simulink model "GS_model"  (R2018b)
settings: Solver=ode5  StartTime=0.0  StopTime=SimuStopTime  FixedStep=T_Simu  RelTol=1e-3
InitFcn:
  | Initial
undefined symbols (not defined in the file or in its folder): Aba10, Aba20, aeroCIP2006_S, aeroCIP2006_X, aeroCIP2006_Y, Agl0, Ass_kS, Ass_n1, Ass_n2, Ass_n3, Ass_n4, Ass_Noise, Ass_R, Ass_Resolution, Ass_TmOrder, AssA_Fix_Abs, AssB_Fix_Abs, AssC_Fix_Abs, AssD_Fix_Abs, AssE_Fix_Aps, AssF_Fix_Aps, C, c_max, c_min, Cd, CenterOfFigNX, CenterOfFigNY, CenterOfFigNZ, CenterOfFigP1, CenterOfFigP2, CenterOfFigPX, CenterOfFigPY, CenterOfFigPZ, Cmu, Crou, DEG2RAD, DiscIntNeverNeededParam, Eg_Dir, Eg_F, Eg_PrepareTime, Eg_r_L_L, Fw_Abf, Fw_Hmax, Fw_J, Fw_Spd0, Fw_Tmax, git_hash_BaseLine, git_hash_Project, Gnss_Noise_Pos, Gnss_Noise_Vel, Gnss_PropgationTime, GyroA_Fix_Abg, GyroA_Noise, GyroB_Fix_Abg, GyroB_Noise, GyroC_Fix_Abg, GyroC_Noise, GyroD_Fix_Abg, GyroD_Noise, h ... (+94)
libraries: simulink x308, sharedutil x46, aerolibutil x37, sharedtransform x31, vrlib x14, aerolibgravity2 x2
(part 14 of 20)

== system GS_model/Subsystem2/Subsystem/Actuator/Magnetorquer/Mt_MathModel/MtA3/Mag_CmdCal/>=<0 to 012 ==
  note: 1--正向
  note: 0
  note: 2--负向
  In1 : Inport
  Add1 : Sum  Inputs=+++
  Cast To Double : DataTypeConversion  OutDataTypeStr=double
  Cast To Double1 : DataTypeConversion  OutDataTypeStr=double
  Cast To Double2 : DataTypeConversion  OutDataTypeStr=double
  Compare To Zero : simulink/Logic and Bit Operations/Compare To Zero  relop=<  OutDataTypeStr=boolean
  Compare To Zero1 : simulink/Logic and Bit Operations/Compare To Zero  relop===  OutDataTypeStr=uint8
  Compare To Zero2 : simulink/Logic and Bit Operations/Compare To Zero  relop=>  OutDataTypeStr=boolean
  Constant1 : Constant
  Constant2 : Constant  Value=0
  Constant20 : Constant  Value=2
  Product1 : Product  SaturateOnIntegerOverflow=on  OutDataTypeStr=Inherit: Same as first input
  Product2 : Product  SaturateOnIntegerOverflow=on  OutDataTypeStr=Inherit: Same as first input
  Product6 : Product  SaturateOnIntegerOverflow=on  OutDataTypeStr=Inherit: Same as first input
  Out1 : Outport
  wires:
  Product1/1 -> Add1/2
  Product6/1 -> Add1/1
  Compare To Zero1/1 -> Cast To Double1/1
  Constant2/1 -> Product1/1
  In1/1 -> Compare To Zero2/1, Compare To Zero1/1, Compare To Zero/1
  Compare To Zero/1 -> Cast To Double/1
  Compare To Zero2/1 -> Cast To Double2/1
  Add1/1 -> Out1/1
  Cast To Double/1 -> Product6/2
  Cast To Double1/1 -> Product1/2
  Constant20/1 -> Product6/1
  Constant1/1 -> Product2/1
  Cast To Double2/1 -> Product2/2
  Product2/1 -> Add1/3

== system GS_model/Subsystem2/Subsystem/Actuator/Magnetorquer/Mt_MathModel/MtA4/Mag_CmdCal/55//AA to +//- ==
  note: 55H:正向
      | AAH:负向
  In1 : Inport
  Add1 : Sum  Inputs=|++
  Cast To Double : DataTypeConversion  OutDataTypeStr=double
  Cast To Double2 : DataTypeConversion  OutDataTypeStr=double
  Compare To Constant : simulink/Logic and Bit Operations/Compare To Constant  relop===  const=85  OutDataTypeStr=boolean
  Compare To Constant1 : simulink/Logic and Bit Operations/Compare To Constant  relop===  const=170  OutDataTypeStr=boolean
  Constant1 : Constant  Value=-1
  Constant20 : Constant
  Product2 : Product  SaturateOnIntegerOverflow=on  OutDataTypeStr=Inherit: Same as first input
  Product6 : Product  SaturateOnIntegerOverflow=on  OutDataTypeStr=Inherit: Same as first input
  Out1 : Outport
  wires:
  Constant1/1 -> Product2/2
  Cast To Double2/1 -> Product2/1
  Product2/1 -> Add1/2
  Constant20/1 -> Product6/1
  Cast To Double/1 -> Product6/2
  Add1/1 -> Out1/1
  Compare To Constant1/1 -> Cast To Double2/1
  Compare To Constant/1 -> Cast To Double/1
  In1/1 -> Compare To Constant1/1, Compare To Constant/1
  Product6/1 -> Add1/1

== system GS_model/Subsystem2/Subsystem/Actuator/Magnetorquer/Mt_MathModel/MtA4/Mag_CmdCal/>=<0 to 012 ==
  note: 2--负向
  note: 0
  note: 1--正向
  In1 : Inport
  Add1 : Sum  Inputs=+++
  Cast To Double : DataTypeConversion  OutDataTypeStr=double
  Cast To Double1 : DataTypeConversion  OutDataTypeStr=double
  Cast To Double2 : DataTypeConversion  OutDataTypeStr=double
  Compare To Zero : simulink/Logic and Bit Operations/Compare To Zero  relop=<  OutDataTypeStr=boolean
  Compare To Zero1 : simulink/Logic and Bit Operations/Compare To Zero  relop===  OutDataTypeStr=uint8
  Compare To Zero2 : simulink/Logic and Bit Operations/Compare To Zero  relop=>  OutDataTypeStr=boolean
  Constant1 : Constant
  Constant2 : Constant  Value=0
  Constant20 : Constant  Value=2
  Product1 : Product  SaturateOnIntegerOverflow=on  OutDataTypeStr=Inherit: Same as first input
  Product2 : Product  SaturateOnIntegerOverflow=on  OutDataTypeStr=Inherit: Same as first input
  Product6 : Product  SaturateOnIntegerOverflow=on  OutDataTypeStr=Inherit: Same as first input
  Out1 : Outport
  wires:
  Product2/1 -> Add1/3
  Cast To Double2/1 -> Product2/2
  Constant1/1 -> Product2/1
  Constant20/1 -> Product6/1
  Cast To Double1/1 -> Product1/2
  Cast To Double/1 -> Product6/2
  Add1/1 -> Out1/1
  Compare To Zero2/1 -> Cast To Double2/1
  Compare To Zero/1 -> Cast To Double/1
  In1/1 -> Compare To Zero/1, Compare To Zero1/1, Compare To Zero2/1
  Constant2/1 -> Product1/1
  Compare To Zero1/1 -> Cast To Double1/1
  Product6/1 -> Add1/1
  Product1/1 -> Add1/2

== system GS_model/Subsystem2/Subsystem/Actuator/Magnetorquer/Mt_MathModel/MtA5/Mag_CmdCal/55//AA to +//- ==
  note: 55H:正向
      | AAH:负向
  In1 : Inport
  Add1 : Sum  Inputs=|++
  Cast To Double : DataTypeConversion  OutDataTypeStr=double
  Cast To Double2 : DataTypeConversion  OutDataTypeStr=double
  Compare To Constant : simulink/Logic and Bit Operations/Compare To Constant  relop===  const=85  OutDataTypeStr=boolean
  Compare To Constant1 : simulink/Logic and Bit Operations/Compare To Constant  relop===  const=170  OutDataTypeStr=boolean
  Constant1 : Constant  Value=-1
  Constant20 : Constant
  Product2 : Product  SaturateOnIntegerOverflow=on  OutDataTypeStr=Inherit: Same as first input
  Product6 : Product  SaturateOnIntegerOverflow=on  OutDataTypeStr=Inherit: Same as first input
  Out1 : Outport
  wires:
  Product6/1 -> Add1/1
  In1/1 -> Compare To Constant/1, Compare To Constant1/1
  Compare To Constant/1 -> Cast To Double/1
  Compare To Constant1/1 -> Cast To Double2/1
  Add1/1 -> Out1/1
  Cast To Double/1 -> Product6/2
  Constant20/1 -> Product6/1
  Product2/1 -> Add1/2
  Cast To Double2/1 -> Product2/1
  Constant1/1 -> Product2/2

== system GS_model/Subsystem2/Subsystem/Actuator/Magnetorquer/Mt_MathModel/MtA5/Mag_CmdCal/>=<0 to 012 ==
  note: 1--正向
  note: 0
  note: 2--负向
  In1 : Inport
  Add1 : Sum  Inputs=+++
  Cast To Double : DataTypeConversion  OutDataTypeStr=double
  Cast To Double1 : DataTypeConversion  OutDataTypeStr=double
  Cast To Double2 : DataTypeConversion  OutDataTypeStr=double
  Compare To Zero : simulink/Logic and Bit Operations/Compare To Zero  relop=<  OutDataTypeStr=boolean
  Compare To Zero1 : simulink/Logic and Bit Operations/Compare To Zero  relop===  OutDataTypeStr=uint8
  Compare To Zero2 : simulink/Logic and Bit Operations/Compare To Zero  relop=>  OutDataTypeStr=boolean
  Constant1 : Constant
  Constant2 : Constant  Value=0
  Constant20 : Constant  Value=2
  Product1 : Product  SaturateOnIntegerOverflow=on  OutDataTypeStr=Inherit: Same as first input
  Product2 : Product  SaturateOnIntegerOverflow=on  OutDataTypeStr=Inherit: Same as first input
  Product6 : Product  SaturateOnIntegerOverflow=on  OutDataTypeStr=Inherit: Same as first input
  Out1 : Outport
  wires:
  Product1/1 -> Add1/2
  Product6/1 -> Add1/1
  Compare To Zero1/1 -> Cast To Double1/1
  Constant2/1 -> Product1/1
  In1/1 -> Compare To Zero2/1, Compare To Zero1/1, Compare To Zero/1
  Compare To Zero/1 -> Cast To Double/1
  Compare To Zero2/1 -> Cast To Double2/1
  Add1/1 -> Out1/1
  Cast To Double/1 -> Product6/2
  Cast To Double1/1 -> Product1/2
  Constant20/1 -> Product6/1
  Constant1/1 -> Product2/1
  Cast To Double2/1 -> Product2/2
  Product2/1 -> Add1/3

== system GS_model/Subsystem2/Subsystem/Actuator/Magnetorquer/Mt_MathModel/MtA6/Mag_CmdCal/55//AA to +//- ==
  note: 55H:正向
      | AAH:负向
  In1 : Inport
  Add1 : Sum  Inputs=|++
  Cast To Double : DataTypeConversion  OutDataTypeStr=double
  Cast To Double2 : DataTypeConversion  OutDataTypeStr=double
  Compare To Constant : simulink/Logic and Bit Operations/Compare To Constant  relop===  const=85  OutDataTypeStr=boolean
  Compare To Constant1 : simulink/Logic and Bit Operations/Compare To Constant  relop===  const=170  OutDataTypeStr=boolean
  Constant1 : Constant  Value=-1
  Constant20 : Constant
  Product2 : Product  SaturateOnIntegerOverflow=on  OutDataTypeStr=Inherit: Same as first input
  Product6 : Product  SaturateOnIntegerOverflow=on  OutDataTypeStr=Inherit: Same as first input
  Out1 : Outport
  wires:
  Constant1/1 -> Product2/2
  Cast To Double2/1 -> Product2/1
  Product2/1 -> Add1/2
  Constant20/1 -> Product6/1
  Cast To Double/1 -> Product6/2
  Add1/1 -> Out1/1
  Compare To Constant1/1 -> Cast To Double2/1
  Compare To Constant/1 -> Cast To Double/1
  In1/1 -> Compare To Constant1/1, Compare To Constant/1
  Product6/1 -> Add1/1

== system GS_model/Subsystem2/Subsystem/Actuator/Magnetorquer/Mt_MathModel/MtA6/Mag_CmdCal/>=<0 to 012 ==
  note: 2--负向
  note: 0
  note: 1--正向
  In1 : Inport
  Add1 : Sum  Inputs=+++
  Cast To Double : DataTypeConversion  OutDataTypeStr=double
  Cast To Double1 : DataTypeConversion  OutDataTypeStr=double
  Cast To Double2 : DataTypeConversion  OutDataTypeStr=double
  Compare To Zero : simulink/Logic and Bit Operations/Compare To Zero  relop=<  OutDataTypeStr=boolean
  Compare To Zero1 : simulink/Logic and Bit Operations/Compare To Zero  relop===  OutDataTypeStr=uint8
  Compare To Zero2 : simulink/Logic and Bit Operations/Compare To Zero  relop=>  OutDataTypeStr=boolean
  Constant1 : Constant
  Constant2 : Constant  Value=0
  Constant20 : Constant  Value=2
  Product1 : Product  SaturateOnIntegerOverflow=on  OutDataTypeStr=Inherit: Same as first input
  Product2 : Product  SaturateOnIntegerOverflow=on  OutDataTypeStr=Inherit: Same as first input
  Product6 : Product  SaturateOnIntegerOverflow=on  OutDataTypeStr=Inherit: Same as first input
  Out1 : Outport
  wires:
  Product2/1 -> Add1/3
  Cast To Double2/1 -> Product2/2
  Constant1/1 -> Product2/1
  Constant20/1 -> Product6/1
  Cast To Double1/1 -> Product1/2
  Cast To Double/1 -> Product6/2
  Add1/1 -> Out1/1
  Compare To Zero2/1 -> Cast To Double2/1
  Compare To Zero/1 -> Cast To Double/1
  In1/1 -> Compare To Zero/1, Compare To Zero1/1, Compare To Zero2/1
  Constant2/1 -> Product1/1
  Compare To Zero1/1 -> Cast To Double1/1
  Product6/1 -> Add1/1
  Product1/1 -> Add1/2

== system GS_model/Subsystem2/Subsystem/PhysicsModel/Environment/Air Torque Subsystem/satalite board/+Y SolarPanel/Compute press of sun radiation1 ==
  note: n
  "Abp " : Inport
  vs(b) : Inport  Port=2
  Fa' : Inport  Port=3
  Abs : Abs
  Dot Product : DotProduct  InputSameDT=on  OutDataTypeStr=Inherit: Inherit via internal rule
  Gain1 : Gain  Gain=S_P1  SaturateOnIntegerOverflow=on  OutDataTypeStr=Inherit: Same as input  ParamDataTypeStr=Inherit: Same as input
  Product1 : Product  Multiplication=Matrix(*)  SaturateOnIntegerOverflow=on  InputSameDT=on  OutDataTypeStr=Inherit: Same as first input
  Product3 : Product  SaturateOnIntegerOverflow=on  OutDataTypeStr=Inherit: Same as first input
  cons : Constant  Value=n_P1P
  "F_panel " : Outport
  wires:
  cons/1 -> Product1/2
  Abs/1 -> Gain1/1
  "Abp "/1 -> Product1/1
  Product1/1 -> Dot Product/2
  Dot Product/1 -> Abs/1
  Gain1/1 -> Product3/1
  Product3/1 -> "F_panel "/1
  Fa'/1 -> Product3/2
  vs(b)/1 -> Dot Product/1

== system GS_model/Subsystem2/Subsystem/PhysicsModel/Environment/Air Torque Subsystem/satalite board/+Y SolarPanel/compute centroi 1 ==
  Cent : Inport
  Abp_PY : Inport  Port=2
  Aba1 : Constant  Value=Aba10  VectorParams1D=off
  Product1 : Product  Multiplication=Matrix(*)  SaturateOnIntegerOverflow=on  InputSameDT=on  OutDataTypeStr=Inherit: Same as first input
  Product12 : Product  Multiplication=Matrix(*)  SaturateOnIntegerOverflow=on  InputSameDT=on  OutDataTypeStr=Inherit: Same as first input
  Sum2 : Sum  Inputs=|+-
  Sum3 : Sum  Inputs=+++  SaturateOnIntegerOverflow=on  InputSameDT=on  OutDataTypeStr=Inherit: Same as first input
  y3 : Constant  Value=CenterOfFigP1  VectorParams1D=off
  ·«°åa°²×°µãÎ»ÖÃ(L) : Constant  Value=r_L_a1_b  VectorParams1D=off
  ·«°åp°²×°µãÎ»ÖÃ(a0) : Constant  Value=r_a1_p1_a1  VectorParams1D=off
  r : Outport
  wires:
  Product12/1 -> Sum3/1
  Aba1/1 -> Product1/1
  ·«°åp°²×°µãÎ»ÖÃ(a0)/1 -> Product1/2
  Product1/1 -> Sum3/2
  y3/1 -> Product12/2
  ·«°åa°²×°µãÎ»ÖÃ(L)/1 -> Sum3/3
  Sum3/1 -> Sum2/1
  Abp_PY/1 -> Product12/1
  Cent/1 -> Sum2/2
  Sum2/1 -> r/1

== system GS_model/Subsystem2/Subsystem/PhysicsModel/Environment/Air Torque Subsystem/satalite board/-Y SolarPanel/Compute press of sun radiation ==
  note: n
  "Abp " : Inport
  vs(b) : Inport  Port=2
  Fa' : Inport  Port=3
  Abs : Abs
  Dot Product : DotProduct  InputSameDT=on  OutDataTypeStr=Inherit: Inherit via internal rule
  Gain1 : Gain  Gain=S_P2  SaturateOnIntegerOverflow=on  OutDataTypeStr=Inherit: Same as input  ParamDataTypeStr=Inherit: Same as input
  Product1 : Product  Multiplication=Matrix(*)  SaturateOnIntegerOverflow=on  InputSameDT=on  OutDataTypeStr=Inherit: Same as first input
  Product3 : Product  SaturateOnIntegerOverflow=on  OutDataTypeStr=Inherit: Same as first input
  cons : Constant  Value=n_P2P
  "F_panel " : Outport
  wires:
  cons/1 -> Product1/2
  Abs/1 -> Gain1/1
  "Abp "/1 -> Product1/1
  Product1/1 -> Dot Product/2
  Dot Product/1 -> Abs/1
  Gain1/1 -> Product3/1
  Product3/1 -> "F_panel "/1
  Fa'/1 -> Product3/2
  vs(b)/1 -> Dot Product/1

== system GS_model/Subsystem2/Subsystem/PhysicsModel/Environment/Air Torque Subsystem/satalite board/-Y SolarPanel/compute centroi 1 ==
  Cent : Inport
  Abp_NY : Inport  Port=2
  Aba1 : Constant  Value=Aba20  VectorParams1D=off
  Product1 : Product  Multiplication=Matrix(*)  SaturateOnIntegerOverflow=on  InputSameDT=on  OutDataTypeStr=Inherit: Same as first input
  Product12 : Product  Multiplication=Matrix(*)  SaturateOnIntegerOverflow=on  InputSameDT=on  OutDataTypeStr=Inherit: Same as first input
  Sum2 : Sum  Inputs=|+-
  Sum3 : Sum  Inputs=+++  SaturateOnIntegerOverflow=on  InputSameDT=on  OutDataTypeStr=Inherit: Same as first input
  y3 : Constant  Value=CenterOfFigP2  VectorParams1D=off
  ·«°åa°²×°µãÎ»ÖÃ(L) : Constant  Value=r_L_a2_b  VectorParams1D=off
  ·«°åp°²×°µãÎ»ÖÃ(a0) : Constant  Value=r_a2_p2_a2  VectorParams1D=off
  r : Outport
  wires:
  Sum2/1 -> r/1
  Cent/1 -> Sum2/2
  Abp_NY/1 -> Product12/1
  Sum3/1 -> Sum2/1
  ·«°åa°²×°µãÎ»ÖÃ(L)/1 -> Sum3/3
  y3/1 -> Product12/2
  Product1/1 -> Sum3/2
  ·«°åp°²×°µãÎ»ÖÃ(a0)/1 -> Product1/2
  Aba1/1 -> Product1/1
  Product12/1 -> Sum3/1

== system GS_model/Subsystem2/Subsystem/PhysicsModel/Environment/Air Torque Subsystem/satalite board/Torque from  board perpendicular to z axis /Compute press of sun radiation ==
  "[Vs]b_nor" : Inport
  Fa' : Inport  Port=2
  Board Orientation : Constant  Value=n_NZ  VectorParams1D=off
  Board Orientation1 : Constant  Value=n_PZ  VectorParams1D=off
  Board Orientation2 : Constant  Value=Szp_board  VectorParams1D=off
  Board Orientation3 : Constant  Value=Szn_board  VectorParams1D=off
  Dot Product : DotProduct  InputSameDT=on  OutDataTypeStr=Inherit: Inherit via internal rule
  Fcn : Fcn  Expr=u(3)
  Product3 : Product  Inputs=3  SaturateOnIntegerOverflow=on  OutDataTypeStr=Inherit: Same as first input
  Switch1 : Switch  SaturateOnIntegerOverflow=on  InputSameDT=on
  Switch2 : Switch  SaturateOnIntegerOverflow=on  InputSameDT=on
  Fz : Outport
  wires:
  Board Orientation1/1 -> Switch2/1
  Board Orientation/1 -> Switch2/3
  Fcn/1 -> Switch2/2
  "[Vs]b_nor"/1 -> Switch1/2, Fcn/1, Dot Product/1
  Switch2/1 -> Dot Product/2
  Product3/1 -> Fz/1
  Dot Product/1 -> Product3/2
  Fa'/1 -> Product3/3
  Board Orientation3/1 -> Switch1/3
  Board Orientation2/1 -> Switch1/1
  Switch1/1 -> Product3/1

== system GS_model/Subsystem2/Subsystem/PhysicsModel/Environment/Air Torque Subsystem/satalite board/Torque from  board perpendicular to z axis /compute centroi 1 ==
  Orientation : Inport
  Cent : Inport  Port=2
  Fcn : Fcn  Expr=u(3)
  Sum2 : Sum  Inputs=|+-
  Switch1 : Switch  SaturateOnIntegerOverflow=on  InputSameDT=on
  y2 : Constant  Value=CenterOfFigNZ  VectorParams1D=off
  y3 : Constant  Value=CenterOfFigPZ  VectorParams1D=off
  r_z : Outport
  wires:
  Sum2/1 -> r_z/1
  y3/1 -> Switch1/1
  y2/1 -> Switch1/3
  Fcn/1 -> Switch1/2
  Orientation/1 -> Fcn/1
  Cent/1 -> Sum2/2
  Switch1/1 -> Sum2/1

== system GS_model/Subsystem2/Subsystem/PhysicsModel/Environment/Air Torque Subsystem/satalite board/Torque from board perpendicular to x axis/Compute press of sun radiation ==
  note: S
  Vs(b) : Inport
  Fa' : Inport  Port=2
  Board Orientation : Constant  Value=n_NX  VectorParams1D=off
  Board Orientation1 : Constant  Value=n_PX  VectorParams1D=off
  Board Orientation2 : Constant  Value=Sx_board  VectorParams1D=off
  Dot Product : DotProduct  InputSameDT=on  OutDataTypeStr=Inherit: Inherit via internal rule
  Fcn : Fcn  Expr=u(1)
  Product3 : Product  Inputs=3  SaturateOnIntegerOverflow=on  OutDataTypeStr=Inherit: Same as first input
  Switch2 : Switch  SaturateOnIntegerOverflow=on  InputSameDT=on
  Fx : Outport
  wires:
  Board Orientation1/1 -> Switch2/1
  Board Orientation/1 -> Switch2/3
  Fcn/1 -> Switch2/2
  Switch2/1 -> Dot Product/2
  Vs(b)/1 -> Fcn/1, Dot Product/1
  Product3/1 -> Fx/1
  Dot Product/1 -> Product3/2
  Board Orientation2/1 -> Product3/1
  Fa'/1 -> Product3/3

== system GS_model/Subsystem2/Subsystem/PhysicsModel/Environment/Air Torque Subsystem/satalite board/Torque from board perpendicular to x axis/compute centroi 1 ==
  Orientation : Inport
  Cent : Inport  Port=2
  Fcn : Fcn  Expr=u(1)
  Sum2 : Sum  Inputs=|+-
  Switch1 : Switch  SaturateOnIntegerOverflow=on  InputSameDT=on
  y2 : Constant  Value=CenterOfFigNX  VectorParams1D=off
  y3 : Constant  Value=CenterOfFigPX  VectorParams1D=off
  r_x : Outport
  wires:
  Sum2/1 -> r_x/1
  y3/1 -> Switch1/1
  y2/1 -> Switch1/3
  Fcn/1 -> Switch1/2
  Orientation/1 -> Fcn/1
  Cent/1 -> Sum2/2
  Switch1/1 -> Sum2/1

== system GS_model/Subsystem2/Subsystem/PhysicsModel/Environment/Air Torque Subsystem/satalite board/Torque from board perpendicular to y axis/Compute press of sun radiation ==
  note: S
  vs(b) : Inport
  Fa' : Inport  Port=2
  Dot Product : DotProduct  InputSameDT=on  OutDataTypeStr=Inherit: Inherit via internal rule
  Fcn : Fcn  Expr=u(2)
  Product1 : Product  Inputs=3  SaturateOnIntegerOverflow=on  OutDataTypeStr=Inherit: Same as first input
  Switch2 : Switch  SaturateOnIntegerOverflow=on  InputSameDT=on
  x1 : Constant  Value=Sy_board  VectorParams1D=off
  x2 : Constant  Value=n_PY  VectorParams1D=off
  x3 : Constant  Value=n_NY  VectorParams1D=off
  Fy : Outport
  wires:
  x2/1 -> Switch2/1
  Fcn/1 -> Switch2/2
  vs(b)/1 -> Fcn/1, Dot Product/1
  Switch2/1 -> Dot Product/2
  Product1/1 -> Fy/1
  Dot Product/1 -> Product1/2
  x1/1 -> Product1/1
  Fa'/1 -> Product1/3
  x3/1 -> Switch2/3

== system GS_model/Subsystem2/Subsystem/PhysicsModel/Environment/Air Torque Subsystem/satalite board/Torque from board perpendicular to y axis/compute centroi 1 ==
  Orientation : Inport
  Cent : Inport  Port=2
  Fcn : Fcn  Expr=u(2)
  Sum2 : Sum  Inputs=|+-
  Switch1 : Switch  SaturateOnIntegerOverflow=on  InputSameDT=on
  y2 : Constant  Value=CenterOfFigNY  VectorParams1D=off
  y3 : Constant  Value=CenterOfFigPY  VectorParams1D=off
  r_y : Outport
  wires:
  Sum2/1 -> r_y/1
  y3/1 -> Switch1/1
  y2/1 -> Switch1/3
  Fcn/1 -> Switch1/2
  Orientation/1 -> Fcn/1
  Cent/1 -> Sum2/2
  Switch1/1 -> Sum2/1

== system GS_model/Subsystem2/Subsystem/PhysicsModel/Environment/Sun  press torque/Sun  press torque2/Sun  press torque/+Y SunPanel ==
  Sun(b) : Inport
  Cent : Inport  Port=2
  Abp : Inport  Port=3
  TC_SunPressCoeff : Inport  Port=4
  3x3 Cross Product : sharedutil/3x3 Cross Product  aMode=aMode
      settings: SourceProductBaseCode=AE,PW,MT,VE,VP
  Compute press of sun radiation : Subsystem  TreatAsAtomicUnit=on
  Product1 : Product  Multiplication=Matrix(*)  SaturateOnIntegerOverflow=on  InputSameDT=on  OutDataTypeStr=Inherit: Same as first input
  Product2 : Product  Multiplication=Matrix(*)  SaturateOnIntegerOverflow=on  InputSameDT=on  OutDataTypeStr=Inherit: Same as first input
  compute centroi 1 : Subsystem  TreatAsAtomicUnit=on
  transpose : Math  Operator=transpose  SaturateOnIntegerOverflow=on
  T : Outport
  F : Outport  Port=2
  wires:
  compute centroi 1/1(r) -> 3x3 Cross Product/1
  Product1/1 -> F/1, 3x3 Cross Product/2
  Compute press of sun radiation/1(F(p)) -> Product1/2
  Product2/1 -> Compute press of sun radiation/1(Sun(p))
  Abp/1 -> compute centroi 1/2(Abp_PY), transpose/1, Product1/1
  Sun(b)/1 -> Product2/2
  transpose/1 -> Product2/1
  Cent/1 -> compute centroi 1/1(Cent)
  3x3 Cross Product/1 -> T/1
  TC_SunPressCoeff/1 -> Compute press of sun radiation/2(TC_SunPressCoeff)

== system GS_model/Subsystem2/Subsystem/PhysicsModel/Environment/Sun  press torque/Sun  press torque2/Sun  press torque/-Y SunPanel ==
  Sun(b) : Inport
  Cent : Inport  Port=2
  Abp : Inport  Port=3
  TC_SunPressCoeff : Inport  Port=4
  3x3 Cross Product : sharedutil/3x3 Cross Product  aMode=aMode
      settings: SourceProductBaseCode=AE,PW,MT,VE,VP
  Compute press of sun radiation : Subsystem  TreatAsAtomicUnit=on
  Product1 : Product  Multiplication=Matrix(*)  SaturateOnIntegerOverflow=on  InputSameDT=on  OutDataTypeStr=Inherit: Same as first input
  Product2 : Product  Multiplication=Matrix(*)  SaturateOnIntegerOverflow=on  InputSameDT=on  OutDataTypeStr=Inherit: Same as first input
  compute centroi 1 : Subsystem  TreatAsAtomicUnit=on
  transpose : Math  Operator=transpose  SaturateOnIntegerOverflow=on
  T : Outport
  F : Outport  Port=2
  wires:
  3x3 Cross Product/1 -> T/1
  Cent/1 -> compute centroi 1/1(Cent)
  transpose/1 -> Product2/1
  Sun(b)/1 -> Product2/2
  Abp/1 -> Product1/1, transpose/1, compute centroi 1/2(Abp_NY)
  Product2/1 -> Compute press of sun radiation/1(Sun(p))
  Compute press of sun radiation/1(F(p)) -> Product1/2
  Product1/1 -> 3x3 Cross Product/2, F/1
  compute centroi 1/1(r) -> 3x3 Cross Product/1
  TC_SunPressCoeff/1 -> Compute press of sun radiation/2(TC_SunPressCoeff)

== system GS_model/Subsystem2/Subsystem/PhysicsModel/Environment/Sun  press torque/Sun  press torque2/Sun  press torque/Torque from   satalite board ==
  SunOrientation : Inport
  Cent : Inport  Port=2
  TC_SunPressCoeff : Inport  Port=3
  Sum : Sum  Inputs=+++
  Sum1 : Sum  Inputs=+++
  "Torque from  board perpendicular to z axis " : Subsystem  TreatAsAtomicUnit=on
  Torque from board perpendicular to x axis : Subsystem  TreatAsAtomicUnit=on
  Torque from board perpendicular to y axis : Subsystem  TreatAsAtomicUnit=on
  T_board : Outport
  F_board : Outport  Port=2
  wires:
  Sum1/1 -> F_board/1
  Sum/1 -> T_board/1
  Torque from board perpendicular to x axis/2(Fx) -> Sum1/1
  Torque from board perpendicular to y axis/2(Fy) -> Sum1/2
  "Torque from  board perpendicular to z axis "/2(Fz) -> Sum1/3
  "Torque from  board perpendicular to z axis "/1(Tz) -> Sum/3
  Torque from board perpendicular to x axis/1(Tx) -> Sum/1
  Torque from board perpendicular to y axis/1(Ty) -> Sum/2
  SunOrientation/1 -> "Torque from  board perpendicular to z axis "/1(Sun Orientation), Torque from board perpendicular to y axis/1(Sun Orientation), Torque from board perpendicular to x axis/1(Sun Orientation)
  Cent/1 -> "Torque from  board perpendicular to z axis "/2(Cent), Torque from board perpendicular to y axis/2(Cent), Torque from board perpendicular to x axis/2(Cent)
  TC_SunPressCoeff/1 -> "Torque from  board perpendicular to z axis "/3(TC_SunPressCoeff), Torque from board perpendicular to y axis/3(TC_SunPressCoeff), Torque from board perpendicular to x axis/3(TC_SunPressCoeff)

== system GS_model/Subsystem2/Subsystem/Sensor/Ass/BodyAss(A&B&C&D)Model/Subsystem/AssErrModel/AssErrSet ==
  note: Switch
  note: Period
  note: AmpCoff
  note: Switch
  note: AmpCoff
  AssCur : Inport
  TC_AssErr_Constant : Inport  Port=2
  TC_AssErr_WildValue : Inport  Port=3
  TC_AssErr_Jump : Inport  Port=4
  TC_StErr_Wave : Inport  Port=5
  AssErrSet_Constant : Subsystem
  AssErrSet_Jump : Subsystem
  AssErrSet_Wave : Subsystem
  AssErrSet_WildValue : Subsystem
  Demux : Demux  Outputs=2
  Demux1 : Demux  Outputs=3
  JumpSet : Constant  Value=0.04
  Terminator : Terminator
  WaveSet : SignalGenerator  WaveForm=square
  WildValueSet : Constant  Value=0.09
  TM_Ass_Cur : Outport
  wires:
  TC_StErr_Wave/1 -> Demux/1
  TC_AssErr_Jump/1 -> Demux1/1
  Demux1/2 -> Terminator/1
  WildValueSet/1 -> AssErrSet_WildValue/2(ErrValue)
  TC_AssErr_WildValue/1 -> AssErrSet_WildValue/3(ErrSwitch)
  TC_AssErr_Constant/1 -> AssErrSet_Constant/1(ErrSwitch)
  AssCur/1 -> AssErrSet_Constant/2(Ass_in)
  AssErrSet_Constant/1(Ass_out) -> AssErrSet_WildValue/1(Ass_in)
  AssErrSet_WildValue/1(Ass_out) -> AssErrSet_Jump/1(Ass_in)
  Demux1/1 -> AssErrSet_Jump/3(ErrSwitch)
  Demux1/3 -> AssErrSet_Jump/4(AssJumpErrAmpCoff)
  JumpSet/1 -> AssErrSet_Jump/2(ErrValue)
  AssErrSet_Jump/1(Ass_out) -> AssErrSet_Wave/1(Ass_in)
  AssErrSet_Wave/1(Ass_out) -> TM_Ass_Cur/1
  WaveSet/1 -> AssErrSet_Wave/2(ErrValue)
  Demux/1 -> AssErrSet_Wave/3(ErrSwitch)
  Demux/2 -> AssErrSet_Wave/4(AssWaveErrAmpCoff)

== system GS_model/Subsystem2/Subsystem/Sensor/Ass/BodyAss(A&B&C&D)Model/Subsystem/AssErrModel/If Action Subsystem ==
  In1 : Inport
  Action Port : ActionPort  ActionType=then
  Out1 : Outport
  wires:
  In1/1 -> Out1/1

== system GS_model/Subsystem2/Subsystem/Sensor/Ass/BodyAss(A&B&C&D)Model/Subsystem/AssErrModel/If Action Subsystem1 ==
  In1 : Inport
  Action Port : ActionPort  ActionType=else
  Out1 : Outport
  wires:
  In1/1 -> Out1/1

== system GS_model/Subsystem2/Subsystem/Sensor/Ass/BodyAss(A&B&C&D)Model/Subsystem/AssErrModel/Triggered Subsystem1 ==
  In1 : Inport
  Enable : EnablePort
  Out1 : Outport  InitialOutput=0
  wires:
  In1/1 -> Out1/1

== system GS_model/Subsystem2/Subsystem/Sensor/Ass/BodyAss(A&B&C&D)Model/Subsystem/AssErrModel/Triggered Subsystem2 ==
  In1 : Inport
  Enable : EnablePort
  Out1 : Outport  InitialOutput=0
  wires:
  In1/1 -> Out1/1

== system GS_model/Subsystem2/Subsystem/Sensor/Ass/BodyAss(A&B&C&D)Model/Subsystem/AssErrModel/Triggered Subsystem3 ==
  In1 : Inport
  Enable : EnablePort
  Out1 : Outport  InitialOutput=0
  wires:
  In1/1 -> Out1/1

== system GS_model/Subsystem2/Subsystem/Sensor/Ass/BodyAss(A&B&C&D)Model/Subsystem/AssErrModel/Triggered Subsystem4 ==
  In1 : Inport
  Enable : EnablePort
  Out1 : Outport  InitialOutput=0
  wires:
  In1/1 -> Out1/1

== system GS_model/Subsystem2/Subsystem/Sensor/Ass/BodyAss(A&B&C&D)Model/Subsystem/AssErrModel/Triggered Subsystem5 ==
  In1 : Inport
  Enable : EnablePort
  Out1 : Outport  InitialOutput=0
  wires:
  In1/1 -> Out1/1

== system GS_model/Subsystem2/Subsystem/Sensor/Ass/BodyAss(A&B&C&D)Model/Subsystem1/AssErrModel/AssErrSet ==
  note: AmpCoff
  note: Switch
  note: AmpCoff
  note: Period
  note: Switch
  AssCur : Inport
  TC_AssErr_Constant : Inport  Port=2
  TC_AssErr_WildValue : Inport  Port=3
  TC_AssErr_Jump : Inport  Port=4
  TC_StErr_Wave : Inport  Port=5
  AssErrSet_Constant : Subsystem
  AssErrSet_Jump : Subsystem
  AssErrSet_Wave : Subsystem
  AssErrSet_WildValue : Subsystem
  Demux : Demux  Outputs=2
  Demux1 : Demux  Outputs=3
  JumpSet : Constant  Value=0.04
  Terminator : Terminator
  WaveSet : SignalGenerator  WaveForm=square
  WildValueSet : Constant  Value=0.09
  TM_Ass_Cur : Outport
  wires:
  Demux/2 -> AssErrSet_Wave/4(AssWaveErrAmpCoff)
  Demux/1 -> AssErrSet_Wave/3(ErrSwitch)
  WaveSet/1 -> AssErrSet_Wave/2(ErrValue)
  AssErrSet_Wave/1(Ass_out) -> TM_Ass_Cur/1
  AssErrSet_Jump/1(Ass_out) -> AssErrSet_Wave/1(Ass_in)
  JumpSet/1 -> AssErrSet_Jump/2(ErrValue)
  Demux1/3 -> AssErrSet_Jump/4(AssJumpErrAmpCoff)
  Demux1/1 -> AssErrSet_Jump/3(ErrSwitch)
  AssErrSet_WildValue/1(Ass_out) -> AssErrSet_Jump/1(Ass_in)
  AssErrSet_Constant/1(Ass_out) -> AssErrSet_WildValue/1(Ass_in)
  AssCur/1 -> AssErrSet_Constant/2(Ass_in)
  TC_AssErr_Constant/1 -> AssErrSet_Constant/1(ErrSwitch)
  TC_AssErr_WildValue/1 -> AssErrSet_WildValue/3(ErrSwitch)
  WildValueSet/1 -> AssErrSet_WildValue/2(ErrValue)
  Demux1/2 -> Terminator/1
  TC_AssErr_Jump/1 -> Demux1/1
  TC_StErr_Wave/1 -> Demux/1

== system GS_model/Subsystem2/Subsystem/Sensor/Ass/BodyAss(A&B&C&D)Model/Subsystem1/AssErrModel/If Action Subsystem ==
  In1 : Inport
  Action Port : ActionPort  ActionType=then
  Out1 : Outport
  wires:
  In1/1 -> Out1/1

== system GS_model/Subsystem2/Subsystem/Sensor/Ass/BodyAss(A&B&C&D)Model/Subsystem1/AssErrModel/If Action Subsystem1 ==
  In1 : Inport
  Action Port : ActionPort  ActionType=else
  Out1 : Outport
  wires:
  In1/1 -> Out1/1

== system GS_model/Subsystem2/Subsystem/Sensor/Ass/BodyAss(A&B&C&D)Model/Subsystem1/AssErrModel/Triggered Subsystem1 ==
  In1 : Inport
  Enable : EnablePort
  Out1 : Outport  InitialOutput=0
  wires:
  In1/1 -> Out1/1

== system GS_model/Subsystem2/Subsystem/Sensor/Ass/BodyAss(A&B&C&D)Model/Subsystem1/AssErrModel/Triggered Subsystem2 ==
  In1 : Inport
  Enable : EnablePort
  Out1 : Outport  InitialOutput=0
  wires:
  In1/1 -> Out1/1

== system GS_model/Subsystem2/Subsystem/Sensor/Ass/BodyAss(A&B&C&D)Model/Subsystem1/AssErrModel/Triggered Subsystem3 ==
  In1 : Inport
  Enable : EnablePort
  Out1 : Outport  InitialOutput=0
  wires:
  In1/1 -> Out1/1

== system GS_model/Subsystem2/Subsystem/Sensor/Ass/BodyAss(A&B&C&D)Model/Subsystem1/AssErrModel/Triggered Subsystem4 ==
  In1 : Inport
  Enable : EnablePort
  Out1 : Outport  InitialOutput=0
  wires:
  In1/1 -> Out1/1

== system GS_model/Subsystem2/Subsystem/Sensor/Ass/BodyAss(A&B&C&D)Model/Subsystem1/AssErrModel/Triggered Subsystem5 ==
  In1 : Inport
  Enable : EnablePort
  Out1 : Outport  InitialOutput=0
  wires:
  In1/1 -> Out1/1

== system GS_model/Subsystem2/Subsystem/Sensor/Ass/BodyAss(A&B&C&D)Model/Subsystem2/AssErrModel/AssErrSet ==
  note: Switch
  note: Period
  note: AmpCoff
  note: Switch
  note: AmpCoff
  AssCur : Inport
  TC_AssErr_Constant : Inport  Port=2
  TC_AssErr_WildValue : Inport  Port=3
  TC_AssErr_Jump : Inport  Port=4
  TC_StErr_Wave : Inport  Port=5
  AssErrSet_Constant : Subsystem
  AssErrSet_Jump : Subsystem
  AssErrSet_Wave : Subsystem
  AssErrSet_WildValue : Subsystem
  Demux : Demux  Outputs=2
  Demux1 : Demux  Outputs=3
  JumpSet : Constant  Value=0.04
  Terminator : Terminator
  WaveSet : SignalGenerator  WaveForm=square
  WildValueSet : Constant  Value=0.09
  TM_Ass_Cur : Outport
  wires:
  TC_StErr_Wave/1 -> Demux/1
  TC_AssErr_Jump/1 -> Demux1/1
  Demux1/2 -> Terminator/1
  WildValueSet/1 -> AssErrSet_WildValue/2(ErrValue)
  TC_AssErr_WildValue/1 -> AssErrSet_WildValue/3(ErrSwitch)
  TC_AssErr_Constant/1 -> AssErrSet_Constant/1(ErrSwitch)
  AssCur/1 -> AssErrSet_Constant/2(Ass_in)
  AssErrSet_Constant/1(Ass_out) -> AssErrSet_WildValue/1(Ass_in)
  AssErrSet_WildValue/1(Ass_out) -> AssErrSet_Jump/1(Ass_in)
  Demux1/1 -> AssErrSet_Jump/3(ErrSwitch)
  Demux1/3 -> AssErrSet_Jump/4(AssJumpErrAmpCoff)
  JumpSet/1 -> AssErrSet_Jump/2(ErrValue)
  AssErrSet_Jump/1(Ass_out) -> AssErrSet_Wave/1(Ass_in)
  AssErrSet_Wave/1(Ass_out) -> TM_Ass_Cur/1
  WaveSet/1 -> AssErrSet_Wave/2(ErrValue)
  Demux/1 -> AssErrSet_Wave/3(ErrSwitch)
  Demux/2 -> AssErrSet_Wave/4(AssWaveErrAmpCoff)

== system GS_model/Subsystem2/Subsystem/Sensor/Ass/BodyAss(A&B&C&D)Model/Subsystem2/AssErrModel/If Action Subsystem ==
  In1 : Inport
  Action Port : ActionPort  ActionType=then
  Out1 : Outport
  wires:
  In1/1 -> Out1/1

== system GS_model/Subsystem2/Subsystem/Sensor/Ass/BodyAss(A&B&C&D)Model/Subsystem2/AssErrModel/If Action Subsystem1 ==
  In1 : Inport
  Action Port : ActionPort  ActionType=else
  Out1 : Outport
  wires:
  In1/1 -> Out1/1

== system GS_model/Subsystem2/Subsystem/Sensor/Ass/BodyAss(A&B&C&D)Model/Subsystem2/AssErrModel/Triggered Subsystem1 ==
  In1 : Inport
  Enable : EnablePort
  Out1 : Outport  InitialOutput=0
  wires:
  In1/1 -> Out1/1

== system GS_model/Subsystem2/Subsystem/Sensor/Ass/BodyAss(A&B&C&D)Model/Subsystem2/AssErrModel/Triggered Subsystem2 ==
  In1 : Inport
  Enable : EnablePort
  Out1 : Outport  InitialOutput=0
  wires:
  In1/1 -> Out1/1

== system GS_model/Subsystem2/Subsystem/Sensor/Ass/BodyAss(A&B&C&D)Model/Subsystem2/AssErrModel/Triggered Subsystem3 ==
  In1 : Inport
  Enable : EnablePort
  Out1 : Outport  InitialOutput=0
  wires:
  In1/1 -> Out1/1

== system GS_model/Subsystem2/Subsystem/Sensor/Ass/BodyAss(A&B&C&D)Model/Subsystem2/AssErrModel/Triggered Subsystem4 ==
  In1 : Inport
  Enable : EnablePort
  Out1 : Outport  InitialOutput=0
  wires:
  In1/1 -> Out1/1

== system GS_model/Subsystem2/Subsystem/Sensor/Ass/BodyAss(A&B&C&D)Model/Subsystem2/AssErrModel/Triggered Subsystem5 ==
  In1 : Inport
  Enable : EnablePort
  Out1 : Outport  InitialOutput=0
  wires:
  In1/1 -> Out1/1

== system GS_model/Subsystem2/Subsystem/Sensor/Ass/BodyAss(A&B&C&D)Model/Subsystem3/AssErrModel/AssErrSet ==
  note: AmpCoff
  note: Switch
  note: AmpCoff
  note: Period
  note: Switch
  AssCur : Inport
  TC_AssErr_Constant : Inport  Port=2
  TC_AssErr_WildValue : Inport  Port=3
  TC_AssErr_Jump : Inport  Port=4
  TC_StErr_Wave : Inport  Port=5
  AssErrSet_Constant : Subsystem
  AssErrSet_Jump : Subsystem
  AssErrSet_Wave : Subsystem
  AssErrSet_WildValue : Subsystem
  Demux : Demux  Outputs=2
  Demux1 : Demux  Outputs=3
  JumpSet : Constant  Value=0.04
  Terminator : Terminator
  WaveSet : SignalGenerator  WaveForm=square
  WildValueSet : Constant  Value=0.09
  TM_Ass_Cur : Outport
  wires:
  Demux/2 -> AssErrSet_Wave/4(AssWaveErrAmpCoff)
  Demux/1 -> AssErrSet_Wave/3(ErrSwitch)
  WaveSet/1 -> AssErrSet_Wave/2(ErrValue)
  AssErrSet_Wave/1(Ass_out) -> TM_Ass_Cur/1
  AssErrSet_Jump/1(Ass_out) -> AssErrSet_Wave/1(Ass_in)
  JumpSet/1 -> AssErrSet_Jump/2(ErrValue)
  Demux1/3 -> AssErrSet_Jump/4(AssJumpErrAmpCoff)
  Demux1/1 -> AssErrSet_Jump/3(ErrSwitch)
  AssErrSet_WildValue/1(Ass_out) -> AssErrSet_Jump/1(Ass_in)
  AssErrSet_Constant/1(Ass_out) -> AssErrSet_WildValue/1(Ass_in)
  AssCur/1 -> AssErrSet_Constant/2(Ass_in)
  TC_AssErr_Constant/1 -> AssErrSet_Constant/1(ErrSwitch)
  TC_AssErr_WildValue/1 -> AssErrSet_WildValue/3(ErrSwitch)
  WildValueSet/1 -> AssErrSet_WildValue/2(ErrValue)
  Demux1/2 -> Terminator/1
  TC_AssErr_Jump/1 -> Demux1/1
  TC_StErr_Wave/1 -> Demux/1

== system GS_model/Subsystem2/Subsystem/Sensor/Ass/BodyAss(A&B&C&D)Model/Subsystem3/AssErrModel/If Action Subsystem ==
  In1 : Inport
  Action Port : ActionPort  ActionType=then
  Out1 : Outport
  wires:
  In1/1 -> Out1/1

== system GS_model/Subsystem2/Subsystem/Sensor/Ass/BodyAss(A&B&C&D)Model/Subsystem3/AssErrModel/If Action Subsystem1 ==
  In1 : Inport
  Action Port : ActionPort  ActionType=else
  Out1 : Outport
  wires:
  In1/1 -> Out1/1

== system GS_model/Subsystem2/Subsystem/Sensor/Ass/BodyAss(A&B&C&D)Model/Subsystem3/AssErrModel/Triggered Subsystem1 ==
  In1 : Inport
  Enable : EnablePort
  Out1 : Outport  InitialOutput=0
  wires:
  In1/1 -> Out1/1

== system GS_model/Subsystem2/Subsystem/Sensor/Ass/BodyAss(A&B&C&D)Model/Subsystem3/AssErrModel/Triggered Subsystem2 ==
  In1 : Inport
  Enable : EnablePort
  Out1 : Outport  InitialOutput=0
  wires:
  In1/1 -> Out1/1

== system GS_model/Subsystem2/Subsystem/Sensor/Ass/BodyAss(A&B&C&D)Model/Subsystem3/AssErrModel/Triggered Subsystem3 ==
  In1 : Inport
  Enable : EnablePort
  Out1 : Outport  InitialOutput=0
  wires:
  In1/1 -> Out1/1

== system GS_model/Subsystem2/Subsystem/Sensor/Ass/BodyAss(A&B&C&D)Model/Subsystem3/AssErrModel/Triggered Subsystem4 ==
  In1 : Inport
  Enable : EnablePort
  Out1 : Outport  InitialOutput=0
  wires:
  In1/1 -> Out1/1

== system GS_model/Subsystem2/Subsystem/Sensor/Ass/BodyAss(A&B&C&D)Model/Subsystem3/AssErrModel/Triggered Subsystem5 ==
  In1 : Inport
  Enable : EnablePort
  Out1 : Outport  InitialOutput=0
  wires:
  In1/1 -> Out1/1

== system GS_model/Subsystem2/Subsystem/Sensor/Ass/SolarPanelAss(E&F)Model/Subsystem/AssErrModel/AssErrSet ==
  note: Switch
  note: Period
  note: AmpCoff
  note: Switch
  note: AmpCoff
  AssCur : Inport
  TC_AssErr_Constant : Inport  Port=2
  TC_AssErr_WildValue : Inport  Port=3
  TC_AssErr_Jump : Inport  Port=4
  TC_StErr_Wave : Inport  Port=5
  AssErrSet_Constant : Subsystem
  AssErrSet_Jump : Subsystem
  AssErrSet_Wave : Subsystem
  AssErrSet_WildValue : Subsystem
  Demux : Demux  Outputs=2
  Demux1 : Demux  Outputs=3
  JumpSet : Constant  Value=0.04
  Terminator : Terminator
  WaveSet : SignalGenerator  WaveForm=square
  WildValueSet : Constant  Value=0.09
  TM_Ass_Cur : Outport
  wires:
  TC_StErr_Wave/1 -> Demux/1
  TC_AssErr_Jump/1 -> Demux1/1
  Demux1/2 -> Terminator/1
  WildValueSet/1 -> AssErrSet_WildValue/2(ErrValue)
  TC_AssErr_WildValue/1 -> AssErrSet_WildValue/3(ErrSwitch)
  TC_AssErr_Constant/1 -> AssErrSet_Constant/1(ErrSwitch)
  AssCur/1 -> AssErrSet_Constant/2(Ass_in)
  AssErrSet_Constant/1(Ass_out) -> AssErrSet_WildValue/1(Ass_in)
  AssErrSet_WildValue/1(Ass_out) -> AssErrSet_Jump/1(Ass_in)
  Demux1/1 -> AssErrSet_Jump/3(ErrSwitch)
  Demux1/3 -> AssErrSet_Jump/4(AssJumpErrAmpCoff)
  JumpSet/1 -> AssErrSet_Jump/2(ErrValue)
  AssErrSet_Jump/1(Ass_out) -> AssErrSet_Wave/1(Ass_in)
  AssErrSet_Wave/1(Ass_out) -> TM_Ass_Cur/1
  WaveSet/1 -> AssErrSet_Wave/2(ErrValue)
  Demux/1 -> AssErrSet_Wave/3(ErrSwitch)
  Demux/2 -> AssErrSet_Wave/4(AssWaveErrAmpCoff)

== system GS_model/Subsystem2/Subsystem/Sensor/Ass/SolarPanelAss(E&F)Model/Subsystem/AssErrModel/If Action Subsystem ==
  In1 : Inport
  Action Port : ActionPort  ActionType=then
  Out1 : Outport
  wires:
  In1/1 -> Out1/1

== system GS_model/Subsystem2/Subsystem/Sensor/Ass/SolarPanelAss(E&F)Model/Subsystem/AssErrModel/If Action Subsystem1 ==
  In1 : Inport
  Action Port : ActionPort  ActionType=else
  Out1 : Outport
  wires:
  In1/1 -> Out1/1

== system GS_model/Subsystem2/Subsystem/Sensor/Ass/SolarPanelAss(E&F)Model/Subsystem/AssErrModel/Triggered Subsystem1 ==
  In1 : Inport
  Enable : EnablePort
  Out1 : Outport  InitialOutput=0
  wires:
  In1/1 -> Out1/1

== system GS_model/Subsystem2/Subsystem/Sensor/Ass/SolarPanelAss(E&F)Model/Subsystem/AssErrModel/Triggered Subsystem2 ==
  In1 : Inport
  Enable : EnablePort
  Out1 : Outport  InitialOutput=0
  wires:
  In1/1 -> Out1/1

== system GS_model/Subsystem2/Subsystem/Sensor/Ass/SolarPanelAss(E&F)Model/Subsystem/AssErrModel/Triggered Subsystem3 ==
  In1 : Inport
  Enable : EnablePort
  Out1 : Outport  InitialOutput=0
  wires:
  In1/1 -> Out1/1

== system GS_model/Subsystem2/Subsystem/Sensor/Ass/SolarPanelAss(E&F)Model/Subsystem/AssErrModel/Triggered Subsystem4 ==
  In1 : Inport
  Enable : EnablePort
  Out1 : Outport  InitialOutput=0
  wires:
  In1/1 -> Out1/1

== system GS_model/Subsystem2/Subsystem/Sensor/Ass/SolarPanelAss(E&F)Model/Subsystem/AssErrModel/Triggered Subsystem5 ==
  In1 : Inport
  Enable : EnablePort
  Out1 : Outport  InitialOutput=0
  wires:
  In1/1 -> Out1/1

== system GS_model/Subsystem2/Subsystem/Sensor/Ass/SolarPanelAss(E&F)Model/Subsystem1/AssErrModel/AssErrSet ==
  note: Switch
  note: Period
  note: AmpCoff
  note: Switch
  note: AmpCoff
  AssCur : Inport
  TC_AssErr_Constant : Inport  Port=2
  TC_AssErr_WildValue : Inport  Port=3
  TC_AssErr_Jump : Inport  Port=4
  TC_StErr_Wave : Inport  Port=5
  AssErrSet_Constant : Subsystem
  AssErrSet_Jump : Subsystem
  AssErrSet_Wave : Subsystem
  AssErrSet_WildValue : Subsystem
  Demux : Demux  Outputs=2
  Demux1 : Demux  Outputs=3
  JumpSet : Constant  Value=0.04
  Terminator : Terminator
  WaveSet : SignalGenerator  WaveForm=square
  WildValueSet : Constant  Value=0.09
  TM_Ass_Cur : Outport
  wires:
  TC_StErr_Wave/1 -> Demux/1
  TC_AssErr_Jump/1 -> Demux1/1
  Demux1/2 -> Terminator/1
  WildValueSet/1 -> AssErrSet_WildValue/2(ErrValue)
  TC_AssErr_WildValue/1 -> AssErrSet_WildValue/3(ErrSwitch)
  TC_AssErr_Constant/1 -> AssErrSet_Constant/1(ErrSwitch)
  AssCur/1 -> AssErrSet_Constant/2(Ass_in)
  AssErrSet_Constant/1(Ass_out) -> AssErrSet_WildValue/1(Ass_in)
  AssErrSet_WildValue/1(Ass_out) -> AssErrSet_Jump/1(Ass_in)
  Demux1/1 -> AssErrSet_Jump/3(ErrSwitch)
  Demux1/3 -> AssErrSet_Jump/4(AssJumpErrAmpCoff)
  JumpSet/1 -> AssErrSet_Jump/2(ErrValue)
  AssErrSet_Jump/1(Ass_out) -> AssErrSet_Wave/1(Ass_in)
  AssErrSet_Wave/1(Ass_out) -> TM_Ass_Cur/1
  WaveSet/1 -> AssErrSet_Wave/2(ErrValue)
  Demux/1 -> AssErrSet_Wave/3(ErrSwitch)
  Demux/2 -> AssErrSet_Wave/4(AssWaveErrAmpCoff)

== system GS_model/Subsystem2/Subsystem/Sensor/Ass/SolarPanelAss(E&F)Model/Subsystem1/AssErrModel/If Action Subsystem ==
  In1 : Inport
  Action Port : ActionPort  ActionType=then
  Out1 : Outport
  wires:
  In1/1 -> Out1/1

== system GS_model/Subsystem2/Subsystem/Sensor/Ass/SolarPanelAss(E&F)Model/Subsystem1/AssErrModel/If Action Subsystem1 ==
  In1 : Inport
  Action Port : ActionPort  ActionType=else
  Out1 : Outport
  wires:
  In1/1 -> Out1/1

== system GS_model/Subsystem2/Subsystem/Sensor/Ass/SolarPanelAss(E&F)Model/Subsystem1/AssErrModel/Triggered Subsystem1 ==
  In1 : Inport
  Enable : EnablePort
  Out1 : Outport  InitialOutput=0
  wires:
  In1/1 -> Out1/1

== system GS_model/Subsystem2/Subsystem/Sensor/Ass/SolarPanelAss(E&F)Model/Subsystem1/AssErrModel/Triggered Subsystem2 ==
  In1 : Inport
  Enable : EnablePort
  Out1 : Outport  InitialOutput=0
  wires:
  In1/1 -> Out1/1

== system GS_model/Subsystem2/Subsystem/Sensor/Ass/SolarPanelAss(E&F)Model/Subsystem1/AssErrModel/Triggered Subsystem3 ==
  In1 : Inport
  Enable : EnablePort
  Out1 : Outport  InitialOutput=0
  wires:
  In1/1 -> Out1/1

== system GS_model/Subsystem2/Subsystem/Sensor/Ass/SolarPanelAss(E&F)Model/Subsystem1/AssErrModel/Triggered Subsystem4 ==
  In1 : Inport
  Enable : EnablePort
  Out1 : Outport  InitialOutput=0
  wires:
  In1/1 -> Out1/1

== system GS_model/Subsystem2/Subsystem/Sensor/Ass/SolarPanelAss(E&F)Model/Subsystem1/AssErrModel/Triggered Subsystem5 ==
  In1 : Inport
  Enable : EnablePort
  Out1 : Outport  InitialOutput=0
  wires:
  In1/1 -> Out1/1

== system GS_model/Subsystem2/Subsystem/Sensor/GNSS/GNSSErrModel/GNSSErrSet_Pos/GNSSErrSet_Constant/Triggered Subsystem1 ==
  In1 : Inport
  Enable : EnablePort
  Out1 : Outport
  wires:
  In1/1 -> Out1/1

== system GS_model/Subsystem2/Subsystem/Sensor/GNSS/GNSSErrModel/GNSSErrSet_Pos/GNSSErrSet_Constant/Triggered Subsystem2 ==
  In1 : Inport
  Enable : EnablePort
  Out1 : Outport
  wires:
  In1/1 -> Out1/1

== system GS_model/Subsystem2/Subsystem/Sensor/GNSS/GNSSErrModel/GNSSErrSet_Pos/GNSSErrSet_Constant/Triggered Subsystem8 ==
  In1 : Inport
  Enable : EnablePort
  Out1 : Outport
  wires:
  In1/1 -> Out1/1

== system GS_model/Subsystem2/Subsystem/Sensor/GNSS/GNSSErrModel/GNSSErrSet_Pos1/GNSSErrSet_Constant/Triggered Subsystem1 ==
  In1 : Inport
  Enable : EnablePort
  Out1 : Outport
  wires:
  In1/1 -> Out1/1

== system GS_model/Subsystem2/Subsystem/Sensor/GNSS/GNSSErrModel/GNSSErrSet_Pos1/GNSSErrSet_Constant/Triggered Subsystem2 ==
  In1 : Inport
  Enable : EnablePort
  Out1 : Outport
  wires:
  In1/1 -> Out1/1

== system GS_model/Subsystem2/Subsystem/Sensor/GNSS/GNSSErrModel/GNSSErrSet_Pos1/GNSSErrSet_Constant/Triggered Subsystem8 ==
  In1 : Inport
  Enable : EnablePort
  Out1 : Outport
  wires:
  In1/1 -> Out1/1

== system GS_model/Subsystem2/Subsystem/Sensor/Gyro/GyroAModel/GyroErrSet/GyroErrSet/GyroErrSet_Constant ==
  w_in : Inport
  ErrSwitch : Inport  Port=2
  Compare To Zero : simulink/Logic and Bit Operations/Compare To Zero  relop===  OutDataTypeStr=boolean
  Compare To Zero1 : simulink/Logic and Bit Operations/Compare To Zero  relop===  OutDataTypeStr=boolean
  Compare To Zero2 : simulink/Logic and Bit Operations/Compare To Zero  relop===  OutDataTypeStr=boolean
  Constant : Constant
  Constant1 : Constant  Value=2
  Constant2 : Constant  Value=3
  Demux : Demux  Outputs=3
  Demux1 : Demux  Outputs=2
  Logical Operator : Logic  Operator=OR  AllPortsSameDT=off  OutDataTypeStr=boolean
  Logical Operator1 : Logic  Operator=OR  AllPortsSameDT=off  OutDataTypeStr=boolean
  Logical Operator2 : Logic  Operator=OR  AllPortsSameDT=off  OutDataTypeStr=boolean
  Memory : Memory
  Memory1 : Memory
  Memory2 : Memory
  Mux : Mux  Inputs=3
  Relational Operator1 : RelationalOperator  Operator===  OutDataTypeStr=boolean  RndMeth=Simplest
  Relational Operator2 : RelationalOperator  Operator===  OutDataTypeStr=boolean  RndMeth=Simplest
  Relational Operator9 : RelationalOperator  Operator===  OutDataTypeStr=boolean  RndMeth=Simplest
  Switch1 : Switch  Criteria=u2 > Threshold  Threshold=0.5
  Switch2 : Switch  Criteria=u2 > Threshold  Threshold=0.5
  Switch3 : Switch  Criteria=u2 > Threshold  Threshold=0.5
  Triggered Subsystem1 : Subsystem  TreatAsAtomicUnit=on
  Triggered Subsystem2 : Subsystem  TreatAsAtomicUnit=on
  Triggered Subsystem8 : Subsystem  TreatAsAtomicUnit=on
  w_out : Outport
  wires:
  w_in/1 -> Demux/1
  Switch1/1 -> Memory/1, Mux/1
  Memory/1 -> Switch1/1
  ErrSwitch/1 -> Demux1/1
  Demux/1 -> Switch1/3
  Demux/2 -> Switch2/3
  Memory1/1 -> Switch2/1
  Switch2/1 -> Mux/2, Memory1/1
  Triggered Subsystem1/1(Out1) -> Switch2/2
  Demux/3 -> Switch3/3
  Memory2/1 -> Switch3/1
  Switch3/1 -> Mux/3, Memory2/1
  Triggered Subsystem2/1(Out1) -> Switch3/2
  Constant/1 -> Relational Operator9/2
  Triggered Subsystem8/1(Out1) -> Switch1/2
  Constant1/1 -> Relational Operator1/2
  Demux1/1 -> Relational Operator9/1, Compare To Zero1/1, Compare To Zero2/1, Relational Operator2/1, Relational Operator1/1, Compare To Zero/1
  Demux1/2 -> Triggered Subsystem8/1(In1), Triggered Subsystem2/1(In1), Triggered Subsystem1/1(In1)
  Constant2/1 -> Relational Operator2/2
  Mux/1 -> w_out/1
  Logical Operator/1 -> Triggered Subsystem8/Enable
  Relational Operator9/1 -> Logical Operator/2
  Compare To Zero/1 -> Logical Operator/1
  Relational Operator1/1 -> Logical Operator1/2
  Logical Operator1/1 -> Triggered Subsystem1/Enable
  Compare To Zero1/1 -> Logical Operator1/1
  Relational Operator2/1 -> Logical Operator2/2
  Compare To Zero2/1 -> Logical Operator2/1
  Logical Operator2/1 -> Triggered Subsystem2/Enable

== system GS_model/Subsystem2/Subsystem/Sensor/Gyro/GyroAModel/GyroErrSet/GyroErrSet/GyroErrSet_Jump ==
  w_in : Inport
  ErrSet : Inport  Port=2
  Add : Sum  Inputs=|++
  Add1 : Sum  Inputs=|++
  Add2 : Sum  Inputs=|++
  Compare To Zero : simulink/Logic and Bit Operations/Compare To Zero  relop===  OutDataTypeStr=boolean
  Compare To Zero1 : simulink/Logic and Bit Operations/Compare To Zero  relop===  OutDataTypeStr=boolean
  Compare To Zero2 : simulink/Logic and Bit Operations/Compare To Zero  relop===  OutDataTypeStr=boolean
  Constant : Constant
  Constant1 : Constant  Value=2
  Constant2 : Constant  Value=3
  Demux : Demux  Outputs=3
  Demux1 : Demux
  JumpSet : Constant  Value=1*DEG2RAD
  Logical Operator : Logic  Operator=OR  AllPortsSameDT=off  OutDataTypeStr=boolean
  Logical Operator1 : Logic  Operator=OR  AllPortsSameDT=off  OutDataTypeStr=boolean
  Logical Operator2 : Logic  Operator=OR  AllPortsSameDT=off  OutDataTypeStr=boolean
  Mux : Mux  Inputs=3
  Product : Product
  Product1 : Product
  Product2 : Product
  Relational Operator1 : RelationalOperator  Operator===  OutDataTypeStr=boolean  RndMeth=Simplest
  Relational Operator2 : RelationalOperator  Operator===  OutDataTypeStr=boolean  RndMeth=Simplest
  Relational Operator5 : RelationalOperator  Operator===  OutDataTypeStr=boolean  RndMeth=Simplest
  Switch1 : Switch  Criteria=u2 > Threshold  Threshold=0.5
  Switch2 : Switch  Criteria=u2 > Threshold  Threshold=0.5
  Switch3 : Switch  Criteria=u2 > Threshold  Threshold=0.5
  Terminator : Terminator
  Triggered Subsystem1 : Subsystem  TreatAsAtomicUnit=on
  Triggered Subsystem2 : Subsystem  TreatAsAtomicUnit=on
  Triggered Subsystem8 : Subsystem  TreatAsAtomicUnit=on
  w_out : Outport
  wires:
  Demux/1 -> Add/2, Switch3/3
  Demux/2 -> Add1/2, Switch1/3
  Add2/1 -> Switch2/1
  Mux/1 -> w_out/1
  Add1/1 -> Switch1/1
  Demux1/2 -> Triggered Subsystem8/1(In1), Triggered Subsystem1/1(In1), Triggered Subsystem2/1(In1)  "Switch"
  Switch3/1 -> Mux/1
  Demux/3 -> Switch2/3, Add2/2
  Add/1 -> Switch3/1
  Demux1/3 -> Terminator/1  "Period"
  Switch1/1 -> Mux/2
  ErrSet/1 -> Demux1/1
  Demux1/4 -> Product2/2, Product1/2, Product/2  "Coff"
  Constant1/1 -> Relational Operator1/2
  Triggered Subsystem2/1(Out1) -> Switch2/2
  Switch2/1 -> Mux/3
  JumpSet/1 -> Product2/1, Product1/1, Product/1
  Triggered Subsystem8/1(Out1) -> Switch3/2
  Constant/1 -> Relational Operator5/2
  Triggered Subsystem1/1(Out1) -> Switch1/2
  w_in/1 -> Demux/1
  Product/1 -> Add/1
  Product1/1 -> Add1/1
  Product2/1 -> Add2/1
  Relational Operator5/1 -> Logical Operator/2
  Logical Operator/1 -> Triggered Subsystem8/Enable
  Compare To Zero/1 -> Logical Operator/1
  Compare To Zero1/1 -> Logical Operator1/1
  Logical Operator1/1 -> Triggered Subsystem1/Enable
  Relational Operator1/1 -> Logical Operator1/2
  Demux1/1 -> Compare To Zero1/1, Relational Operator1/1, Compare To Zero2/1, Relational Operator2/1, Relational Operator5/1, Compare To Zero/1
  Relational Operator2/1 -> Logical Operator2/2
  Logical Operator2/1 -> Triggered Subsystem2/Enable
  Compare To Zero2/1 -> Logical Operator2/1
  Constant2/1 -> Relational Operator2/2
